simulink model "sis_com_red_adelanto"  (R2020b)
settings: Solver=VariableStepAuto  StartTime=0.0  StopTime=4  RelTol=1e-3
settings Model: Creator=carma  LastModifiedBy=carma

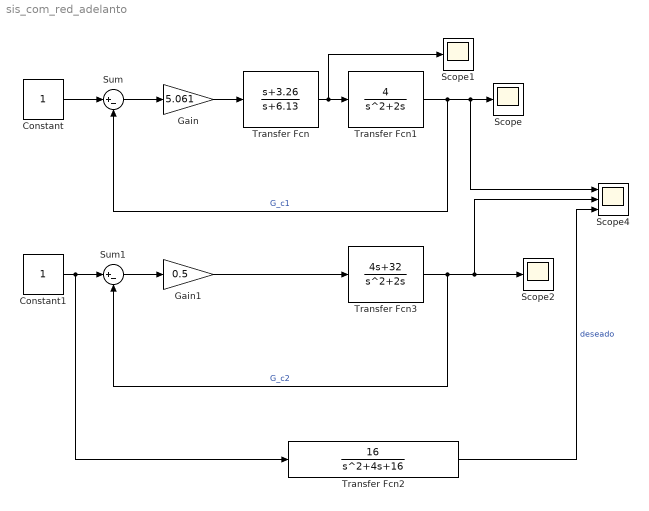
== system sis_com_red_adelanto ==
  Constant : Constant  VectorParams1D=off  SampleTime=-1
  Constant1 : Constant  VectorParams1D=off  SampleTime=-1
  Gain : Gain  Gain=5.061
  Gain1 : Gain  Gain=0.5
  Scope : Scope
  Scope1 : Scope
  Scope2 : Scope
  Scope4 : Scope  NumInputPorts=3
  Sum : Sum  Inputs=|+-
  Sum1 : Sum  Inputs=|+-
  Transfer Fcn : TransferFcn  Numerator=[1 3.26]  Denominator=[1 6.13]
  Transfer Fcn1 : TransferFcn  Numerator=[4]  Denominator=[1 2 0]
  Transfer Fcn2 : TransferFcn  Numerator=[16]  Denominator=[1 4 16]
  Transfer Fcn3 : TransferFcn  Numerator=[4 32]  Denominator=[1 2 0]
  wires:
  Constant/1 -> Sum/1
  Sum/1 -> Gain/1
  Gain/1 -> Transfer Fcn/1
  Transfer Fcn/1 -> Scope1/1, Transfer Fcn1/1
  Transfer Fcn1/1 -> Scope4/1, Scope/1, Sum/2  "G_c1"
  Transfer Fcn3/1 -> Scope4/2, Scope2/1, Sum1/2  "G_c2"
  Gain1/1 -> Transfer Fcn3/1
  Sum1/1 -> Gain1/1
  Constant1/1 -> Transfer Fcn2/1, Sum1/1
  Transfer Fcn2/1 -> Scope4/3  "deseado"
